simulink model "Feedback_1"  (R2016b)
settings: Solver=VariableStepAuto  StartTime=0.0  StopTime=10000  RelTol=1e-3
libraries: simulink x1
settings Model: Creator=黄天  LastModifiedBy=XuanjieXiao

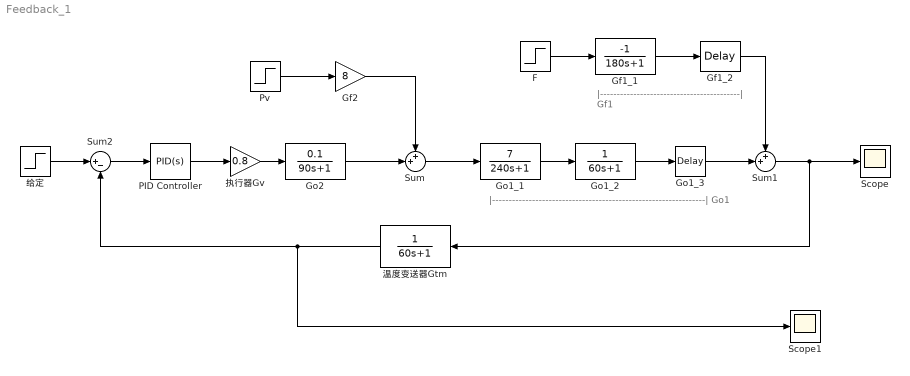
== system Feedback_1 ==
  note: |----------------------------------------------------------------|
      | Go1
  note: |------------------------------------------|
      | Gf1
  F : Step  Time=7500  SampleTime=0
  Gf1_1 : TransferFcn  Numerator=[-1]  Denominator=[180 1]
  Gf1_2 : TransportDelay  DelayTime=180
  Gf2 : Gain  Gain=8
  Go1_1 : TransferFcn  Numerator=[7]  Denominator=[240 1]
  Go1_2 : TransferFcn  Denominator=[60 1]
  Go1_3 : TransportDelay  DelayTime=60
  Go2 : TransferFcn  Numerator=[0.1]  Denominator=[90 1]
  PID Controller : simulink/Continuous/PID Controller  Controller=PID  TimeDomain=Continuous-time  SampleTime=-1  IntegratorMethod=Forward Euler  FilterMethod=Forward Euler  Form=Parallel  UseFilter=on  ControllerParametersSource=internal  P=0.83  I=0.00255  D=0  N=1  InitialConditionSource=internal  InitialConditionForIntegrator=0  InitialConditionForFilter=0  ExternalReset=none  LimitOutput=off  UpperSaturationLimit=inf  LowerSaturationLimit=-inf  LinearizeAsGain=on  AntiWindupMode=none  Kb=1  TrackingMode=off  Kt=1  PParamMin=[]  PParamMax=[]  IParamMin=[]  IParamMax=[]  DParamMin=[]  DParamMax=[]  NParamMin=[]  NParamMax=[]  KbParamMin=[]  KbParamMax=[]  KtParamMin=[]  KtParamMax=[]  POutMin=[]  POutMax=[]  IOutMin=[]  IOutMax=[]  DOutMin=[]  DOutMax=[]  NOutMin=[]  NOutMax=[]  KbOutMin=[]  KbOutMax=[]  KtOutMin=[]  KtOutMax=[]  IntegratorOutMin=[]  IntegratorOutMax=[]  FilterOutMin=[]  FilterOutMax=[]  SumOutMin=[]  SumOutMax=[]  SumI1OutMin=[]  SumI1OutMax=[]  SumI2OutMin=[]  SumI2OutMax=[]  SumI3OutMin=[]  SumI3OutMax=[]  SumDOutMin=[]  SumDOutMax=[]  SaturationOutMin=[]  SaturationOutMax=[]  IntegratorContinuousStateAttributes=''  IntegratorStateMustResolveToSignalObject=off  IntegratorRTWStateStorageClass=Auto  FilterContinuousStateAttributes=''  FilterStateMustResolveToSignalObject=off  FilterRTWStateStorageClass=Auto  DifferentiatorICPrevScaledInput=0  DifferentiatorOutMin=[]  DifferentiatorOutMax=[]
  Pv : Step  Time=3000  SampleTime=0
  Scope : Scope
  Scope1 : Scope
  Sum : Sum  Inputs=++|
  Sum1 : Sum  Inputs=++|
  Sum2 : Sum  Inputs=|+-
  执行器Gv : Gain  Gain=0.8
  温度变送器Gtm : TransferFcn  Denominator=[60 1]
  给定 : Step  After=10  SampleTime=0
  wires:
  Go1_2/1 -> Go1_3/1
  Go1_1/1 -> Go1_2/1
  Gf1_1/1 -> Gf1_2/1
  Go1_3/1 -> Sum1/2
  Sum/1 -> Go1_1/1
  Sum1/1 -> 温度变送器Gtm/1, Scope/1
  温度变送器Gtm/1 -> Scope1/1, Sum2/2
  给定/1 -> Sum2/1
  Go2/1 -> Sum/2
  执行器Gv/1 -> Go2/1
  Sum2/1 -> PID Controller/1
  PID Controller/1 -> 执行器Gv/1
  F/1 -> Gf1_1/1
  Gf1_2/1 -> Sum1/1
  Pv/1 -> Gf2/1
  Gf2/1 -> Sum/1
